simulink model "FPGA_Comm_test_control"  (Simulink 7.6)
settings: Solver=ode4  StartTime=0.0  StopTime=500  FixedStep=0.01  MaxStep=1e-1  RelTol=1e-3
values from neighbouring files (symbols this model uses):
  s1 = op1(1)    [fpu_test.m]
settings Model: Creator=jordan  LastModifiedBy=jordan
settings GRTTargetCC: ExtMode=on

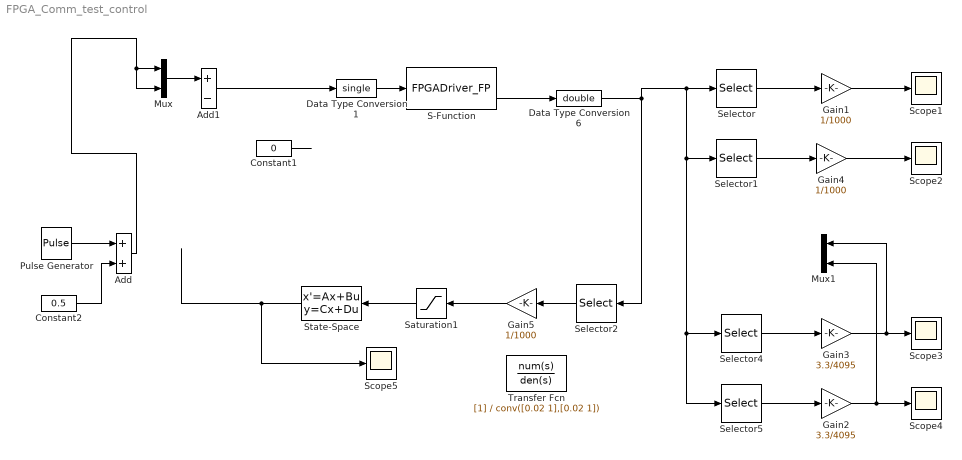
== system FPGA_Comm_test_control ==
  Add : Sum
  Add1 : Sum  Inputs=+-  SampleTime=0.01
  Constant1 : Constant  Value=0
  Constant2 : Constant  Value=0.5
  Data Type Conversion1 : DataTypeConversion  OutDataTypeStr=single
  Data Type Conversion6 : DataTypeConversion  OutDataTypeStr=double
  Gain1 : Gain  Gain=1/1000
  Gain2 : Gain  Gain=3.3/4095
  Gain3 : Gain  Gain=3.3/4095
  Gain4 : Gain  Gain=1/1000
  Gain5 : Gain  Gain=1/1000
  Mux : Mux  Inputs=2
  Mux1 : Mux  Inputs=2
  Pulse Generator : DiscretePulseGenerator  PulseType=Time based  Amplitude=0.5  Period=20  PulseWidth=50
  S-Function : S-Function  FunctionName=FPGADriver_FP  EnableBusSupport=off
  Saturation1 : Saturate  UpperLimit=5  LowerLimit=-5  LinearizeAsGain=off  RndMeth=Nearest
  Scope{1..5} (5 alike) : Scope
      Scope1 settings: TimeRange=50  YMin=-0.9  YMax=1  MaxDataPoints=50000
      Scope2 settings: TimeRange=50  YMin=-0.3  YMax=1.5  MaxDataPoints=50000
      Scope3 settings: TimeRange=50  YMin=5.55112e-017  YMax=1.5  SaveName=ScopeData2  MaxDataPoints=50000
      Scope4 settings: TimeRange=50  YMin=2.77556e-017  YMax=1.05  SaveName=ScopeData3  MaxDataPoints=50000
      Scope5 settings: TimeRange=50  YMin=-7  YMax=3.5  SaveName=ScopeData4  MaxDataPoints=50000
  Selector : Selector  InputPortWidth=4  IndexOptions=Index vector (dialog)  Indices=1  OutputSizes=1
  Selector1 : Selector  InputPortWidth=4  IndexOptions=Index vector (dialog)  Indices=2  OutputSizes=1
  Selector2 : Selector  InputPortWidth=4  IndexOptions=Index vector (dialog)  Indices=[1 2]  OutputSizes=1
  Selector4 : Selector  InputPortWidth=4  IndexOptions=Index vector (dialog)  Indices=3  OutputSizes=1
  Selector5 : Selector  InputPortWidth=4  IndexOptions=Index vector (dialog)  Indices=4  OutputSizes=1
  State-Space : StateSpace  A=s1.a  B=s1.b  C=s1.c  D=s1.d
  Transfer Fcn : TransferFcn  Denominator=conv([0.02 1],[0.02 1])
  wires:
  S-Function/2 -> Data Type Conversion6/1
  Data Type Conversion1/1 -> S-Function/1
  Data Type Conversion6/1 -> Selector/1, Selector1/1, Selector4/1, Selector5/1, Selector2/1
  Mux/1 -> Add1/1
  Selector/1 -> Gain1/1
  Pulse Generator/1 -> Add/1
  Constant2/1 -> Add/2
  Constant1/1 -> ?
  Selector1/1 -> Gain4/1
  Selector4/1 -> Gain3/1
  Selector5/1 -> Gain2/1
  Gain2/1 -> Scope4/1, Mux1/2
  Add1/1 -> Data Type Conversion1/1
  Gain3/1 -> Scope3/1, Mux1/1
  Gain1/1 -> Scope1/1
  Gain4/1 -> Scope2/1
  Selector2/1 -> Gain5/1
  State-Space/1 -> Scope5/1
  Saturation1/1 -> State-Space/1
  Gain5/1 -> Saturation1/1
  Add/1 -> Mux/2, Mux/1
